simulink model "debug_simulink10e1"  (R2020a)
settings: Solver=ode23t  StartTime=0.0  StopTime=1000  MaxStep=1e-4  RelTol=1e-3
undefined symbols (not defined in the file): parameter
libraries: nesl_utility x5, fl_lib x3, ee_lib x2, simulink x2, dspsigops x2, aerolibanimutils x1, powerlib_meascontrol x1
settings Model: Creator=ibrahim yosry  LastModifiedBy=ibrahim yosry
settings SolverCC: InitialStep=1e-4

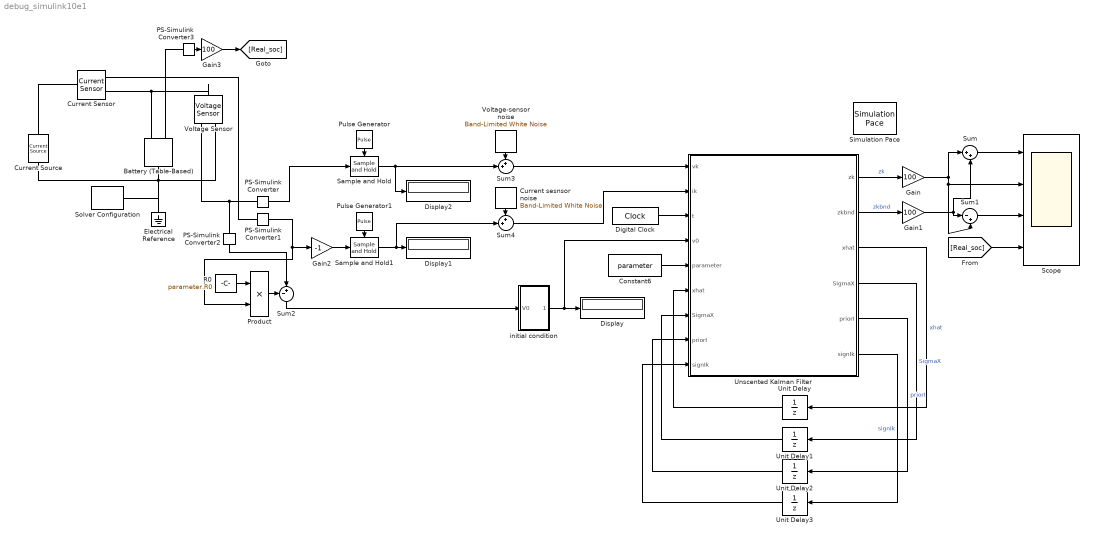
== system debug_simulink10e1 ==
  Battery (Table-Based) : ee_lib/Sources/Battery (Table-Based)  SOC_vec=parameter.soc  T_dependence=ee.enum.temperature_dependence.no  T_vec=[273.15, 298.15, 323.15] K  V0_mat=[3.2, 3.1, 3.14; 3.25, 3.27, 3.3; 3.28, 3.31, 3.34; 3.33, 3.5, 3.59] V  V0_vec=parameter.ocv V  R0_mat=[.03, .015, .002; .04, .017, .008; .039, .012, .006; .027, .013, .021] Ohm  R0_vec=parameter.R0*ones(length(parameter.soc),1) Ohm  AH_vec=[2.9, 4.1, 4.2] hr*A  AH=parameter.Q hr*A  prm_leak=ee.enum.battery.prm_leak.disabled  Rleak_vec=[8000, 7000, 6000] Ohm  Rleak=7e3 Ohm  extrapolation_option=ee.enum.extrapolation.nearest  prm_dyn=ee.enum.battery.prm_dyn.rc1  R1_mat=[.089, .076, .01; .042, .022, .099; .019, .007, .002; .051, .043, .029] Ohm  R1_vec=parameter.R*ones(length(parameter.soc),1) Ohm  tau1_mat=[44, 148, 235; 93, 110, 1000; 19, 27, 133; .5, 22, 3] s  tau1_vec=parameter.RC*ones(length(parameter.soc),1) s  R2_mat=[.014, .382, .407; .028, .006, .007; .014, .007, .006; .333, .956, .912] Ohm  R2_vec=[.382, .006, .007, .956] Ohm  tau2_mat=[1, 44, 5644; 11, 24, 506; 2, 14, 330; 3310, 13419, 30216] s  tau2_vec=[44, 24, 14, 13419] s  R3_mat=[.014, .382, .407; .028, .006, .007; .014, .007, .006; .333, .956, .912] Ohm  R3_vec=[.382, .006, .007, .956] Ohm  tau3_mat=[1, 44, 5644; 11, 24, 506; 2, 14, 330; 3310, 13419, 30216] s  tau3_vec=[44, 24, 14, 13419] s  R4_mat=[.014, .382, .407; .028, .006, .007; .014, .007, .006; .333, .956, .912] Ohm  R4_vec=[.382, .006, .007, .956] Ohm  tau4_mat=[1, 44, 5644; 11, 24, 506; 2, 14, 330; 3310, 13419, 30216] s  tau4_vec=[44, 24, 14, 13419] s  R5_mat=[.014, .382, .407; .028, .006, .007; .014, .007, .006; .333, .956, .912] Ohm  R5_vec=[.382, .006, .007, .956] Ohm  tau5_mat=[1, 44, 5644; 11, 24, 506; 2, 14, 330; 3310, 13419, 30216] s  tau5_vec=[44, 24, 14, 13419] s  prm_fade=ee.enum.battery.prm_fade.equations  N0=100  dV0=0  dR0=0  dAH=0  dRleak=0  dR1=0  dR2=0  dR3=0  dR4=0  dR5=0  N0vec=[100, 200, 300]  Tfadevec=[298.15, 323.15] K  dV0vec=[0, 0, 0]  dR0vec=[0, 0, 0]  dAHvec=[0, 0, 0]  dRleakvec=[0, 0, 0]  dR1vec=[0, 0, 0]  dR2vec=[0, 0, 0]  dR3vec=[0, 0, 0]  dR4vec=[0, 0, 0]  dR5vec=[0, 0, 0]  dV0mat=[0, 0; 0, 0; 0, 0]  dR0mat=[0, 0; 0, 0; 0, 0]  dAHmat=[0, 0; 0, 0; 0, 0]  dRleakmat=[0, 0; 0, 0; 0, 0]  dR1mat=[0, 0; 0, 0; 0, 0]  dR2mat=[0, 0; 0, 0; 0, 0]  dR3mat=[0, 0; 0, 0; 0, 0]  dR4mat=[0, 0; 0, 0; 0, 0]  dR5mat=[0, 0; 0, 0; 0, 0]  temperature=298.15 K  i_specify=off  i_priority=None  i=0 A  i_nominal_specify=off  i_nominal_unit=A  i_nominal_value=1  v_specify=off  v_priority=None  v=0 V  v_nominal_specify=off  v_nominal_unit=V  v_nominal_value=1  stateOfCharge_specify=on  stateOfCharge_priority=High  stateOfCharge=0.183064516129032  stateOfCharge_nominal_specify=off  stateOfCharge_nominal_unit=1  stateOfCharge_nominal_value=1  num_cycles_specify=off  num_cycles_priority=High  num_cycles=0  num_cycles_nominal_specify=off  num_cycles_nominal_unit=1  num_cycles_nominal_value=1  thermal_mass=30000 J/K  temperature_specify=off  temperature_priority=High  temperature_nominal_specify=off  temperature_nominal_unit=K  temperature_nominal_value=1
      settings: SourceProductBaseCode=PS  InternalSimscapePortConfiguration="{\"Bottom\":[],\"Left\":[{\"id\":\"p\",\"label\":\"+\",\"type\":\"foundation.electrical.electrical\"},{\"id\":\"soc\",\"label\":\"SOC\",\"type\":\"output\"}],\"Right\":[{\"id\":\"n\",\"label\":\"-\",\"type\":\"foundation.electrical.electrical\"}],\"Top\":[]}"
  Constant6 : Constant  Value=parameter  VectorParams1D=off  OutDataTypeStr=Bus: parameter_bus  SampleTime=1e-1
  Current Sensor : fl_lib/Electrical/Electrical Sensors/Current Sensor
      settings: SourceProductBaseCode=MT,SS
  Current Source : ee_lib/Sources/Current Source  dc_current=2.9 A  ac_current=0 A  ac_shift=0 rad  ac_frequency=60 Hz  noise_mode=0  PSD=0 A^2/Hz  repeatability=1  auto_seed=2775893241  user_seed=0  sample_time=1e-3 s  i_specify=off  i_priority=None  i=0 A  i_nominal_specify=off  i_nominal_unit=A  i_nominal_value=1  v_specify=off  v_priority=None  v=0 V  v_nominal_specify=off  v_nominal_unit=V  v_nominal_value=1
      settings: SourceProductBaseCode=PS
  Current sesnsor noise : simulink/Sources/Band-Limited White Noise  Cov=[0.001]  Ts=1e-1  seed=[23341]
  Digital Clock : DigitalClock  SampleTime=1e-1
  Display : Display
  Display1 : Display
  Display2 : Display
  Electrical Reference : fl_lib/Electrical/Electrical Elements/Electrical Reference
  Gain : Gain  Gain=100
  Gain1 : Gain  Gain=100
  Gain2 : Gain  Gain=-1
  Gain3 : Gain  Gain=100
  PS-Simulink Converter{,1..3} (4 alike) : nesl_utility/PS-Simulink Converter  PhysicalDomain=network_engine_domain  SubClassName=ps_output  LeftPortType=input  RightPortType=output  PseudoPeriodic=off  Frequencies=[]  Unit=inherit  AffineConversion=off
  Product : Product
  Pulse Generator : DiscretePulseGenerator  PulseType=Time based  Period=1e-1  PulseWidth=5
  Pulse Generator1 : DiscretePulseGenerator  PulseType=Time based  Period=1e-1  PulseWidth=5
  R0 : Constant  Value=parameter.R0  SampleTime=1e-1
  Sample and Hold : dspsigops/Sample and Hold  trig=Rising edge  initCond=0  latchinput=off
  Sample and Hold1 : dspsigops/Sample and Hold  trig=Rising edge  initCond=0  latchinput=off
  Scope : Scope  NumInputPorts=4
  Simulation Pace : aerolibanimutils/Simulation Pace  SimulationPace=100  SleepMode=Auto  OutputPaceError=off  SampleTime=1e-1
  Solver Configuration : nesl_utility/Solver Configuration  PhysicalDomain=network_engine_domain  SubClassName=solver  LeftPortType=input  RightPortType=generic  Tones=[]  Harmonics=[]  SimulateNoise=off  Profile=off  UseLocalSampling=off  EnableSwitchedLinearOptims=on  FrequencyDomain=off  UseCCode=off  RelTol=0.001  AbsTol=1e-06  MinStep=1e-09  ToWorkspace=off  RevertToSquareIcSolve=off  NumHomotopyIterations=100  PhasorMode=off  PhasorModeNumHarmonics=1  DoDC=off  ResidualTolerance=1e-09  UseLocalSolver=off  LocalSolverChoice=NE_BACKWARD_EULER_ADVANCER  LocalSolverSampleTime=1e-4  DoFixedCost=off  MaxNonlinIter=3  MaxModeIter=2  LinearAlgebra=auto  EquationFormulation=NE_TIME_EF  DelaysMemoryBudget=1024  AutomaticFiltering=on  FilteringTimeConstant=0.001  PartitionStorageMethod=AS_NEEDED  PartitionMemoryBudget=1024  PartitionMethod=ROBUST
  Sum : Sum  Inputs=|++
  Sum1 : Sum  Inputs=|-+
  Sum2 : Sum  Inputs=-+|
  Sum3 : Sum  Inputs=++|
  Sum4 : Sum  Inputs=++|
  Unit Delay : UnitDelay  InitialCondition=[1;0;0]  SampleTime=1e-1  HasFrameUpgradeWarning=on
  Unit Delay1 : UnitDelay  InitialCondition=diag([1e-6 1e-8 2e-4])  SampleTime=1e-1  HasFrameUpgradeWarning=on
  Unit Delay2 : UnitDelay  SampleTime=1e-1  HasFrameUpgradeWarning=on
  Unit Delay3 : UnitDelay  SampleTime=1e-1  HasFrameUpgradeWarning=on
  Unscented Kalman Filter : MATLAB Function  TreatAsAtomicUnit=on
  Voltage Sensor : fl_lib/Electrical/Electrical Sensors/Voltage Sensor
      settings: SourceProductBaseCode=MT,SS
  Voltage-sensor noise : simulink/Sources/Band-Limited White Noise  Cov=[0.001]  Ts=1e-1  seed=[23341]
  initial condition : Subsystem
      mask Display: image('F:\hima\zpEWIvRg.jpg'); % Use "Edit Image" on toolstrip to change.
  wires:
  Unscented Kalman Filter/3(xhat) -> Unit Delay/1  "xhat"
  Unscented Kalman Filter/1(zk) -> Gain/1  "zk"
  Unscented Kalman Filter/2(zkbnd) -> Gain1/1  "zkbnd"
  Gain1/1 -> Sum/2, Sum1/1
  Gain/1 -> Sum/1, Sum1/2, Scope/2
  Sum/1 -> Scope/1
  Sum1/1 -> Scope/3
  initial condition/1(Out1) -> Display/1, Unscented Kalman Filter/4(v0)
  Unit Delay/1 -> Unscented Kalman Filter/6("xhat ")
  Pulse Generator/1 -> Sample and Hold/Trigger
  PS-Simulink Converter/1 -> Sample and Hold/1
  Pulse Generator1/1 -> Sample and Hold1/Trigger
  Sample and Hold1/1 -> Sum4/2, Display1/1
  Constant6/1 -> Unscented Kalman Filter/5(parameter)
  Digital Clock/1 -> Unscented Kalman Filter/3(t)
  Unscented Kalman Filter/4(SigmaX) -> Unit Delay1/1  "SigmaX"
  Unscented Kalman Filter/5(priorI) -> Unit Delay2/1  "priorI"
  Unscented Kalman Filter/6(signIk) -> Unit Delay3/1  "signIk"
  Unit Delay3/1 -> Unscented Kalman Filter/9("signIk ")
  Unit Delay2/1 -> Unscented Kalman Filter/8("priorI ")
  Unit Delay1/1 -> Unscented Kalman Filter/7("SigmaX ")
  PS-Simulink Converter1/1 -> Product/2, Gain2/1
  Gain2/1 -> Sample and Hold1/1
  R0/1 -> Product/1
  Product/1 -> Sum2/1
  PS-Simulink Converter2/1 -> Sum2/2
  Sum2/1 -> initial condition/1(V0)
  [Real_soc] -> Scope/4
  PS-Simulink Converter3/1 -> Gain3/1
  Gain3/1 -> [Real_soc]
  Voltage-sensor noise/1 -> Sum3/1
  Sample and Hold/1 -> Display2/1, Sum3/2
  Sum3/1 -> Unscented Kalman Filter/1(vk)
  Current sesnsor noise/1 -> Sum4/1
  Sum4/1 -> Unscented Kalman Filter/2(ik)
  connections:
  Voltage Sensor/LConn1 -- Current Sensor/RConn2 -- Battery (Table-Based)/LConn1
  Voltage Sensor/RConn2 -- Battery (Table-Based)/RConn1 -- Solver Configuration/RConn1 -- Electrical Reference/LConn1 -- Current Source/RConn1
  PS-Simulink Converter/LConn1 -- PS-Simulink Converter2/LConn1 -- Voltage Sensor/RConn1
  Current Sensor/LConn1 -- Current Source/LConn1
  PS-Simulink Converter1/LConn1 -- Current Sensor/RConn1
  PS-Simulink Converter3/LConn1 -- Battery (Table-Based)/LConn2

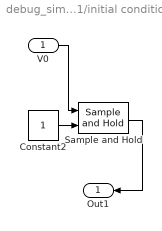
== system debug_simulink10e1/initial condition ==
  V0 : Inport
  Constant2 : Constant  SampleTime=1e-1
  Sample and Hold : powerlib_meascontrol/Additional Components/Sample and Hold  ic=0  Ts=6000000
      settings: SourceProductBaseCode=PS
  Out1 : Outport  VectorParamsAs1DForOutWhenUnconnected=off
  wires:
  Constant2/1 -> Sample and Hold/2
  V0/1 -> Sample and Hold/1
  Sample and Hold/1 -> Out1/1

== matlab function debug_simulink10e1/Unscented Kalman Filter ==
  settings: updateMethod=DISCRETE  sampleTime=1e-1
  data: vk input; zk output; ik input; t input; v0 input; parameter input; xhat input; zkbnd output; xhat output; SigmaX input; priorI input; signIk input; SigmaX output; priorI output; signIk output
function [zk,zkbnd,xhat,SigmaX,priorI,signIk] = iterSPKF(vk,ik,t,v0,parameter,xhat,SigmaX,priorI,signIk)
parameter.deltat=1e-1;
SigmaX0 = diag([1e-6 1e-8 2e-4]);
SigmaV = 2e-1;
SigmaW = 2e-1;
Snoise = chol(blkdiag(SigmaW,SigmaV),'lower');
irk0 = 0;
hk0 = 0;
zkInd = 1;
irkInd = 2;
hkInd = 3;
ocv=parameter.ocv;
soc=parameter.soc;
Nx = 3;
Nw = 1;
Nv = 1;
Na = Nx+Nw+Nv;
h = sqrt(3);
alpha1 = (h*h-Na)/(h*h);
alpha2 = 1/(2*h*h);
alpham = [alpha1; alpha2*ones(2*Na,1)];
alphac = alpham;
RC      = parameter.RC;
G       = parameter.G;
Q       = parameter.Q;
deltat  = parameter.deltat;
R0      = parameter.R0;
R       = parameter.R;
M0      = parameter.M0;
M       = parameter.M;
zkInd   = parameter.zkInd;
irkInd  = parameter.irkInd;
hkInd   = parameter.hkInd;

eta     = 1;
if ik<0 
ik=ik*eta;
end

if t<1e-4
j1=find(min(abs(ocv-v0))==abs(ocv-v0));
j=j1(1,:);
SOC0 = soc(j);
xhat = [SOC0;irk0;hk0];
SigmaX = SigmaX0;
priorI = 0;
signIk = 0;
end

I       =  priorI;
if abs(ik)>Q/100
signIk = sign(ik);
end
xhata = [xhat; zeros([Nw+Nv 1])];
sigmaXa = chol(SigmaX,'lower');
sigmaXa= blkdiag(sigmaXa,Snoise);
Xa = xhata(:,ones([1 2*Na+1])) + h*[zeros([Na 1]),sigmaXa,-sigmaXa];
Xx = stateEqn(Xa(1:Nx,:),I,Xa(Nx+1:Nx+Nw,:),parameter);
xhat = Xx*alpham;
Xs = Xx - xhat(:,ones([1 2*Na+1]));
SigmaX = Xs*diag(alphac)*Xs';
I = ik;
yk = vk;
Y = outputEqn(Xx,I,Xa(5,:),signIk,parameter);
yhat = Y*alpham;
Ys = Y - yhat(:,ones([1 2*Na+1]));
SigmaXY = Xs*diag(alphac)*Ys';
SigmaY = Ys*diag(alphac)*Ys';
L = SigmaXY/SigmaY;
ytelda = yk - yhat;
xhat = xhat + L*ytelda;
xhat(hkInd) = min(0.99,max(-0.99,xhat(hkInd)));
SigmaX = SigmaX - L*SigmaY*L';
priorI = ik;
zk = xhat(zkInd);
zkbnd = 3*sqrt(SigmaX(zkInd,zkInd));
function xnew = stateEqn(xold,current,xnoise,parameter)
current = current + xnoise;
RC      = parameter.RC;
G       = parameter.G;
Q       = parameter.Q;
deltat  = parameter.deltat;
zkInd   = parameter.zkInd;
irkInd  = parameter.irkInd;
hkInd   = parameter.hkInd;
Ah = exp(-abs(current*G*deltat/(3600*Q)));
xnew = 0*xold;
xnew(irkInd,:) = RC*xold(irkInd,:) + (1-RC)*current;
xnew(hkInd,:) = Ah.*xold(hkInd,:) + (Ah-1).*sign(current);
xnew(zkInd,:) = xold(zkInd,:) - current*deltat/(3600*Q);
end
function y = outputEqn(x,current,ynoise,signIk,parameter)
soc     = parameter.soc;
ocv     = parameter.ocv;
R0      = parameter.R0;
R       = parameter.R;
M0      = parameter.M0;
M       = parameter.M;
zkInd   = parameter.zkInd;
irkInd  = parameter.irkInd;
hkInd   = parameter.hkInd;
i=zeros(11,1);
for k=1:11
i2=find(min(abs(soc-x(zkInd,k)*ones(length(soc),1)))==abs(soc-x(zkInd,k)*ones(length(soc),1))); %1241>>length
i(k,1)=i2(1,1);
end
y = ocv(i)' - R * x(irkInd,:) - R0 * current + M * x(hkInd,:) + M0 * signIk + ynoise;
end
end
